simulink model "plant_5_1"  (R2025b)
settings: Solver=VariableStepAuto  StartTime=0.0  StopTime=7  RelTol=1e-3
settings Model: Creator=sengu  LastModifiedBy=sengu

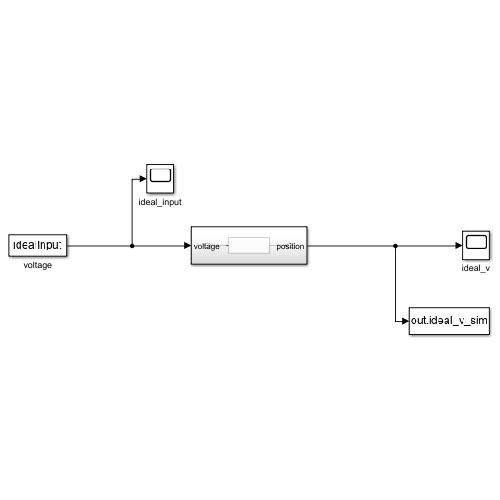
[thumbnail: Simulink's stored preview of the top-level diagram]
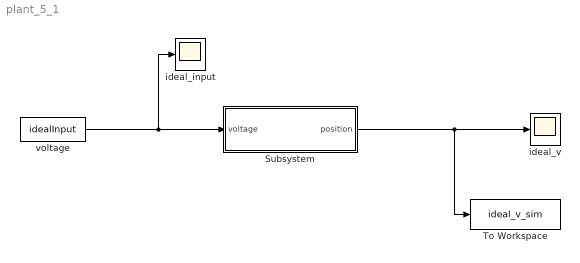
== system plant_5_1 ==
  Subsystem : Subsystem
  To Workspace : ToWorkspace  VariableName=ideal_v_sim  SaveFormat=Timeseries  SampleTime=-1
  ideal_input : Scope
      settings: ActiveDisplayYMinimum=-1  ActiveDisplayYMaximum=1
  ideal_v : Scope
      settings: ActiveDisplayYMinimum=-647.60864284240529  ActiveDisplayYMaximum=623.44679848402507
  voltage : FromWorkspace  VariableName=idealInput  SampleTime=-1
  wires:
  Subsystem/1(position) -> To Workspace/1, ideal_v/1
  voltage/1 -> ideal_input/1, Subsystem/1(voltage)

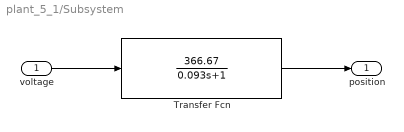
== system plant_5_1/Subsystem ==
  voltage : Inport
  Transfer Fcn : TransferFcn  Numerator=[366.67]  Denominator=[0.093 1]
  position : Outport
  wires:
  voltage/1 -> Transfer Fcn/1
  Transfer Fcn/1 -> position/1
